simulink model "WPTwithMOTOR"  (R2021a)
settings: Solver=FixedStepDiscrete  StartTime=0.0  StopTime=Tfinal  FixedStep=SampleTime  RelTol=1e-3
InitFcn:
  | param
values from neighbouring files (symbols this model uses):
  Cp = 28.5e-9    (= 2.85e-08)    [param.m]
  Cs = 115e-9    (= 1.15e-07)    [param.m]
  ESRA = 1e-7    (= 1e-07)    [param.m]
  J = 0.001    [param.m]
  Lmotor = 1e-3    (= 0.001)    [param.m]
  Lp = 205e-6    (= 0.000205)    [param.m]
  Ls = 51e-6    (= 5.1e-05)    [param.m]
  M = 41e-6    (= 4.1e-05)    [param.m]
  RL = 40    [param.m]
  Rmotor = 2    [param.m]
  SampleTime = 1e-9    (= 1e-09)    [param.m]
  Tfinal = 0.1    [param.m]
  TL = 5    [param.m]
  VDC = 100    [param.m]
undefined symbols (not defined in the file or in its folder): ESLA
libraries: spsSeriesRLCBranchLib x13, spsVoltageMeasurementLib x10, spsCurrentMeasurementLib x10, spsMosfetLib x4, eeStairGenerator x3, spsFourierLib x2, spsDCVoltageSourceLib x1, spsDCMachineLib x1, spsTriangleGeneratorLib x1, spsVariableResistorLib x1, spspowerguiLib x1
settings Model: Creator=enes_  LastModifiedBy=enes_
settings SolverCC: AlgebraicLoopSolver=TrustRegion
settings DataIOCC: ReturnWorkspaceOutputs=off
settings DebuggingCC: SFMachineParentedDataDiag=warning  ArithmeticOperatorsInVariantConditions=warning
settings SFSimCC: SimUseLocalCustomCode=off  CustomCodeUndefinedFunction=UseInterfaceOnly
settings RTWCC: RTWUseLocalCustomCode=off

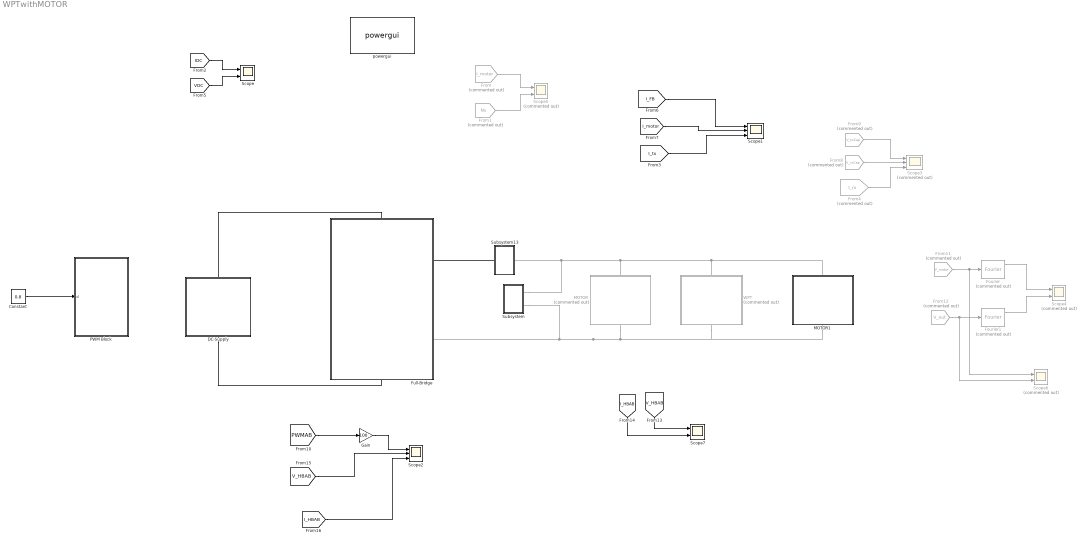
== system WPTwithMOTOR ==
  Constant : Constant  Value=0.8
  DC-Supply : Subsystem
  Fourier : spsFourierLib/Fourier  Commented=on  Freq=80e3  n=1  InInit=[0, 0]  Ts=SampleTime
      settings: SourceProductBaseCode=PS
  Fourier1 : spsFourierLib/Fourier  Commented=on  Freq=80e3  n=1  InInit=[0, 0]  Ts=SampleTime
      settings: SourceProductBaseCode=PS
  From : From  Commented=on  GotoTag=I_motor  TagVisibility=global
  From1 : From  Commented=on  GotoTag=Ns  TagVisibility=global
  From11 : From  Commented=on  GotoTag=V_motor  TagVisibility=global
  From12 : From  Commented=on  GotoTag=V_out  TagVisibility=global
  From4 : From  Commented=on  GotoTag=I_rx  TagVisibility=global
  From8 : From  Commented=on  GotoTag=V_rxCap  TagVisibility=global
  From9 : From  Commented=on  GotoTag=V_txCap  TagVisibility=global
  Full-Bridge : Subsystem
      settings: PortSchema="{\"entries\":[{\"content\":{\"sides\":[{\"content\":{\"connectorIds\":[]},\"type\":\"ConnectorPlacement.EquallySpacedRectSide\",\"uuid\":\"92c2640b-bb56-47f8-9c41-2323b38839f8\"},{\"content\":{\"connectorIds\":[\"RConn1\",\"RConn2\"],\"side\":\"RIGHT\"},\"type\":\"ConnectorPlacement.EquallySpacedRectSide\",\"uuid\":\"0b5c90a1-e2e1-4478-84c9-834496a6568e\"},{\"content\":{\"connectorIds\":[\"LConn1\"],\"side\":\"TOP\"},\"type\":\"ConnectorPlacement.EquallySpacedRectSide\",\"uuid\":\"1c803fb0-9096-4a7d-b495-aabd35d72306\"},{\"content\":{\"connectorIds\":[\"RConn3\"],\"side\":\"BOTTOM\"},\"type\":\"ConnectorPlacement.EquallySpacedRectSide\",\"uuid\":\"5a2d766c-8c3f-4943-ab0f-0e1988e2f8d8\"},{\"content\":{\"connectorIds\":[],\"side\":\"HIDDEN\"},\"type\":\"ConnectorPlacement.EquallySpacedRectSide\",\"uuid\":\"8868c32c-a67f-4887-a91d-dc24242eaee2\"}]},\"type\":\"ConnectorPlacement.EquallySpacedConnector\",\"uuid\":\"a3546067-6216-40b0-bae0-9d71271c5112\"}],\"packageUris\":[\"http://schema.mathworks.com/mf0/Connector/R2020b\"],\"version\":\"1.0\"}"
  Gain : Gain  Gain=100
  MOTOR : Subsystem  Commented=on
  MOTOR1 : Subsystem
  PWM Block : Subsystem
  Scope : Scope  NumInputPorts=2
  Scope1 : Scope  NumInputPorts=3
  Scope2 : Scope  NumInputPorts=3
  Scope3 : Scope  Commented=on  NumInputPorts=3
  Scope4 : Scope  Commented=on  NumInputPorts=2
  Scope5 : Scope  Commented=on  NumInputPorts=2
  Scope6 : Scope  Commented=on  NumInputPorts=2
  Scope7 : Scope  NumInputPorts=2
  Subsystem : Subsystem
  Subsystem13 : Subsystem
  WPT : Subsystem  Commented=on
  powergui : spspowerguiLib/powergui  Priority=1  SimulationMode=Discrete  SampleTime=SampleTime  frequency=60  Iterations=50  frequencyindice=0  Pbase=100e6  ErrMax=1e-4  UnitsV=kV  UnitsW=MW  buscounter=0  FunctionMessages=off  echomessages=off  EnableUseOfTLC=off  CurrentSourceSwitches=off  DisableSnubberDevices=off  DisableRonSwitches=off  DisableVfSwitches=off  DisplayEquations=off  AutomaticDiscreteSolvers=off  SolverType=Tustin/Backward Euler (TBE)  Interpol=off  ExternalGateDelay=off  methode=off  Ts=100  x0status=blocks  SPID=on  SwTol=0  HookPort=off  NonlinearTolerance=1e-4  nMaxIteration=100  ContinueOnMaxIteration=off  RestoreLinks=warning  ResistiveCurrentMeasurement=off  Frange=[1e3:1e3:240e3]  Ylog=off  Xlog=on  ShowGrid=off  save=off  variable=ZData  structure=inputVoltage  ZoomFFT=off  StartTime=0.0  cycles=100  DisplayStyle=1  fundamental=80000  FreqAxis=off  MaxFrequency=240e3  frequencyindicesteady=1  RmsSteady=1  display=off
  wires:
  [IDC] -> Scope/1
  [VDC] -> Scope/2
  From/1 -> Scope5/1
  From1/1 -> Scope5/2
  [I_FB] -> Scope1/1
  [I_motor] -> Scope1/2
  [I_tx] -> Scope1/3
  From9/1 -> Scope3/1
  From8/1 -> Scope3/2
  From4/1 -> Scope3/3
  From11/1 -> Scope6/1, Fourier/1
  From12/1 -> Scope6/2, Fourier1/1
  Fourier/1 -> Scope4/1
  Fourier1/1 -> Scope4/2
  Constant/1 -> PWM Block/1(d)
  [V_HBAB] -> Scope7/1
  [I_HBAB] -> Scope7/2
  [PWMAB] -> Gain/1
  [V_HBAB] -> Scope2/2
  Gain/1 -> Scope2/1
  [I_HBAB] -> Scope2/3
  connections:
  WPT/LConn1 -- Subsystem13/LConn1 -- Subsystem/LConn1 -- MOTOR/LConn1 -- MOTOR1/LConn1
  MOTOR/RConn1 -- Full-Bridge/RConn2 -- Subsystem/LConn2 -- WPT/RConn1 -- MOTOR1/RConn1
  Subsystem13/RConn1 -- Full-Bridge/RConn1
  DC-Supply/LConn1 -- Full-Bridge/LConn1
  DC-Supply/RConn1 -- Full-Bridge/RConn3

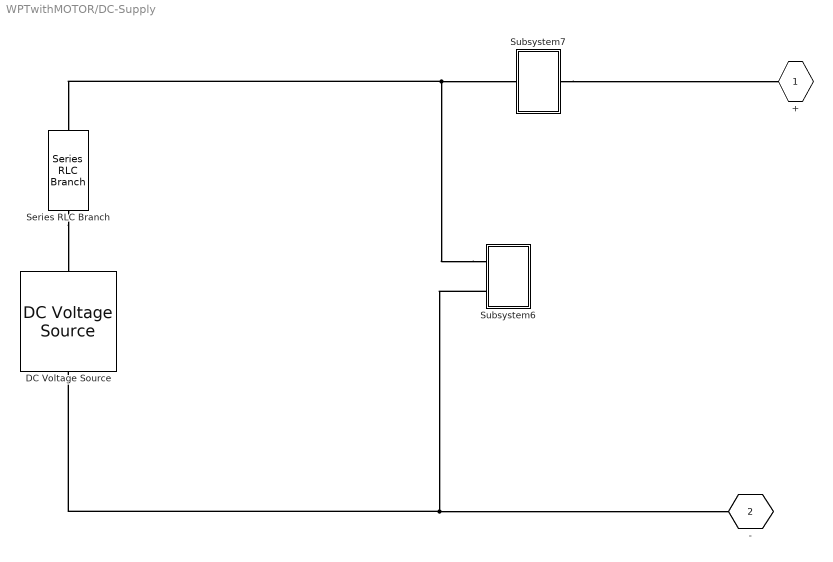
== system WPTwithMOTOR/DC-Supply ==
  DC Voltage Source : spsDCVoltageSourceLib/DC Voltage Source  Amplitude=VDC  Measurements=None
  Series RLC Branch : spsSeriesRLCBranchLib/Series RLC Branch  LConnTagsString=__new0  RConnTagsString=__new0  BranchType=RL  Resistance=1e-3  Inductance=1e-7  SetiL0=off  InitialCurrent=0  Capacitance=1e-6  Setx0=off  InitialVoltage=0  Measurements=None
  Subsystem6 : Subsystem
  Subsystem7 : Subsystem
  + : PMIOPort  Side=Left
  - : PMIOPort  Port=2  Side=Right
  connections:
  Subsystem6/LConn2 -- DC Voltage Source/LConn1 -- -/RConn1
  Subsystem6/LConn1 -- Series RLC Branch/LConn1 -- Subsystem7/RConn1
  Subsystem7/LConn1 -- +/RConn1
  Series RLC Branch/RConn1 -- DC Voltage Source/RConn1

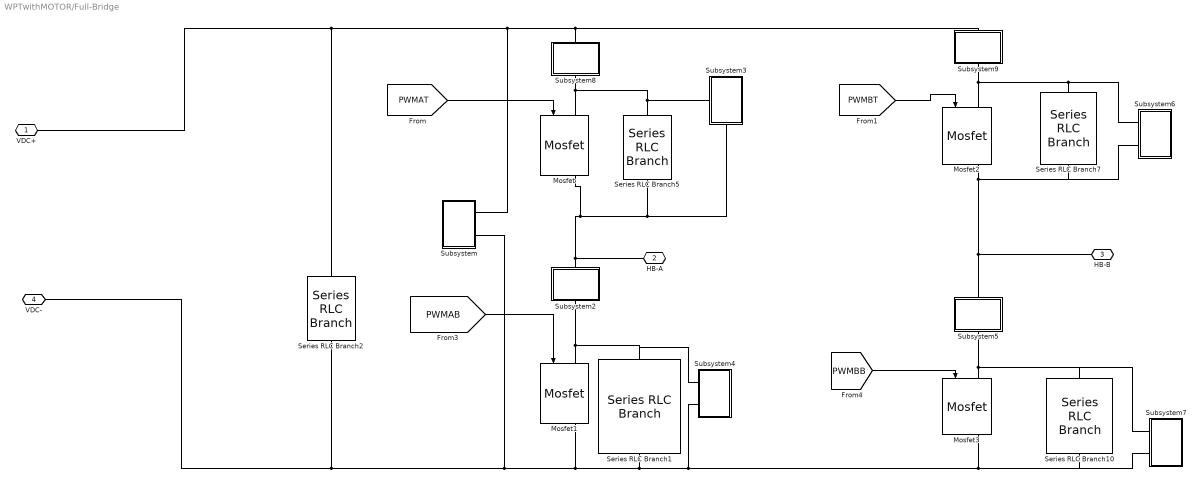
== system WPTwithMOTOR/Full-Bridge ==
  Mosfet{,1..3} (4 alike) : spsMosfetLib/Mosfet  Ron=0.1  Lon=0  Rd=0.01  Vfd=0  IC=0  Rs=1e5  Cs=inf  Measurements=on
  Series RLC Branch{1,5,7,10} (4 alike) : spsSeriesRLCBranchLib/Series RLC Branch  LConnTagsString=__new0  RConnTagsString=__new0  BranchType=C  Resistance=ESRA  Inductance=ESLA  SetiL0=off  InitialCurrent=0  Capacitance=10e-9  Setx0=off  InitialVoltage=0  Measurements=None
  Series RLC Branch2 : spsSeriesRLCBranchLib/Series RLC Branch  LConnTagsString=__new0  RConnTagsString=__new0  BranchType=C  Resistance=ESRA  Inductance=ESLA  SetiL0=off  InitialCurrent=0  Capacitance=100e-3  Setx0=off  InitialVoltage=0  Measurements=None
  Subsystem : Subsystem
  Subsystem2 : Subsystem
  Subsystem3 : Subsystem
      settings: PortSchema="{\"entries\":[{\"content\":{\"sides\":[{\"content\":{\"connectorIds\":[\"LConn1\"]},\"type\":\"ConnectorPlacement.EquallySpacedRectSide\",\"uuid\":\"5fd3471b-77c4-4add-974d-2088884e4e8f\"},{\"content\":{\"connectorIds\":[],\"side\":\"RIGHT\"},\"type\":\"ConnectorPlacement.EquallySpacedRectSide\",\"uuid\":\"3ed3d87c-239d-4488-bb47-dd20adb66433\"},{\"content\":{\"connectorIds\":[],\"side\":\"TOP\"},\"type\":\"ConnectorPlacement.EquallySpacedRectSide\",\"uuid\":\"7d1a83a5-f952-4011-a8a9-3e03fc6b2605\"},{\"content\":{\"connectorIds\":[\"RConn1\"],\"side\":\"BOTTOM\"},\"type\":\"ConnectorPlacement.EquallySpacedRectSide\",\"uuid\":\"37159049-9de9-498e-a62d-c9d42e905d7f\"}]},\"type\":\"ConnectorPlacement.EquallySpacedConnector\",\"uuid\":\"187da425-f362-4fb5-84e5-b88eb8acd0b2\"}],\"packageUris\":[\"http://schema.mathworks.com/mf0/Connector/R2020b\"],\"version\":\"1.0\"}"
  Subsystem4 : Subsystem
  Subsystem5 : Subsystem
  Subsystem6 : Subsystem
  Subsystem7 : Subsystem
  Subsystem8 : Subsystem
  Subsystem9 : Subsystem
  VDC+ : PMIOPort  Side=Left
  HB-A : PMIOPort  Port=2  Side=Right
  HB-B : PMIOPort  Port=3  Side=Right
  VDC- : PMIOPort  Port=4  Side=Right
  wires:
  [PWMAB] -> Mosfet1/1
  [PWMAT] -> Mosfet/1
  [PWMBB] -> Mosfet3/1
  [PWMBT] -> Mosfet2/1
  connections:
  Mosfet1/LConn1 -- Subsystem2/LConn1 -- Subsystem4/LConn1 -- Series RLC Branch1/LConn1
  Subsystem9/LConn1 -- Subsystem6/LConn1 -- Series RLC Branch7/LConn1 -- Mosfet2/LConn1
  VDC+/RConn1 -- Series RLC Branch2/LConn1 -- Subsystem/LConn1 -- Subsystem8/RConn1 -- Subsystem9/RConn1
  Series RLC Branch5/LConn1 -- Subsystem8/LConn1 -- Mosfet/LConn1 -- Subsystem3/LConn1
  VDC-/RConn1 -- Series RLC Branch2/RConn1 -- Subsystem/LConn2 -- Subsystem4/LConn2 -- Subsystem7/LConn2 -- Series RLC Branch10/RConn1 -- Mosfet3/RConn1 -- Series RLC Branch1/RConn1 -- Mosfet1/RConn1
  Subsystem6/LConn2 -- Series RLC Branch7/RConn1 -- HB-B/RConn1 -- Subsystem5/RConn1 -- Mosfet2/RConn1
  Subsystem3/RConn1 -- HB-A/RConn1 -- Subsystem2/RConn1 -- Mosfet/RConn1 -- Series RLC Branch5/RConn1
  Mosfet3/LConn1 -- Subsystem5/LConn1 -- Subsystem7/LConn1 -- Series RLC Branch10/LConn1

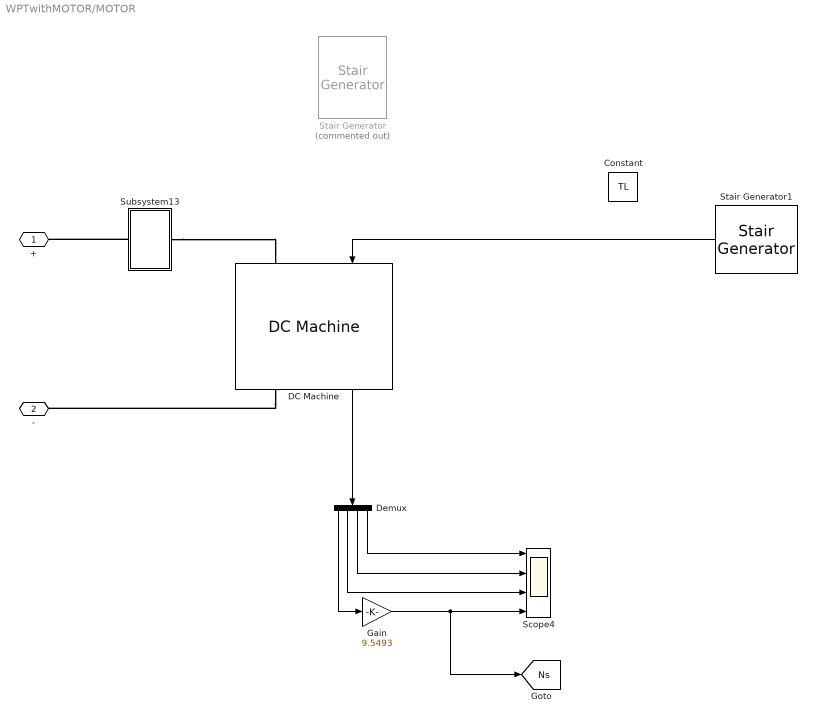
== system WPTwithMOTOR/MOTOR ==
  Constant : Constant  Value=TL
  DC Machine : spsDCMachineLib/DC Machine  PresetModel=No  MechanicalLoad=Torque TL  FieldType=Permanent magnet  ShowDetailedParameters=on  MeasurementBus=off  RLa="[ Rmotor  Lmotor]"  RLf="[ 240  120]"  Laf=1.8  MachineConstant=Back-emf constant (V/rpm)  Ke=Kf  Kt=1.8  J=J  Bm=Bm  Tf=Tf  w0=w0  Ifinit=1  TsPowergui=0  TsBlock=-1
  Demux : Demux
  Gain : Gain  Gain=9.5493
  Scope4 : Scope  NumInputPorts=4
  Stair Generator : eeStairGenerator/Stair Generator  Commented=on  LabelModeActiveChoice=Discrete  TimeInput=Tfinal*[0 1/3 2/3]  AmplitudeInput=TL*[0 1 1/2 ]  SampleTime=-1  RepeatPattern=off  OutDataTypeStr=double
      settings: SourceProductBaseCode=PS
  Stair Generator1 : eeStairGenerator/Stair Generator  LabelModeActiveChoice=Discrete  TimeInput=Tfinal*[0 1/4 2/4 3/4 ]  AmplitudeInput="TL*[1  0.5  1  0.6 ]"  SampleTime=SampleTime  RepeatPattern=off  OutDataTypeStr=double
      settings: SourceProductBaseCode=PS
  Subsystem13 : Subsystem
  + : PMIOPort  Side=Left
  - : PMIOPort  Port=2  Side=Right
  tag scope: Ns=global
  wires:
  Demux/2 -> Scope4/3
  Gain/1 -> [Ns], Scope4/4
  Demux/3 -> Scope4/2
  Demux/1 -> Gain/1
  Demux/4 -> Scope4/1
  DC Machine/1 -> Demux/1
  Stair Generator1/1 -> DC Machine/1
  connections:
  DC Machine/RConn1 -- -/RConn1
  Subsystem13/LConn1 -- DC Machine/LConn1
  Subsystem13/RConn1 -- +/RConn1

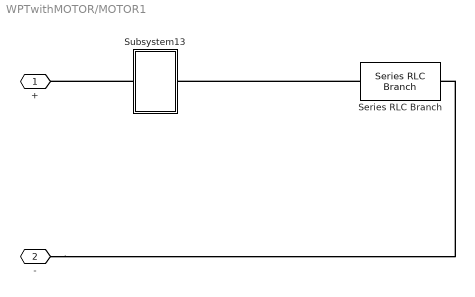
== system WPTwithMOTOR/MOTOR1 ==
  Series RLC Branch : spsSeriesRLCBranchLib/Series RLC Branch  LConnTagsString=__new0  RConnTagsString=__new0  BranchType=RL  Resistance=5  Inductance=7e-3  SetiL0=off  InitialCurrent=0  Capacitance=1e-6  Setx0=off  InitialVoltage=0  Measurements=None
  Subsystem13 : Subsystem
  + : PMIOPort  Side=Left
  - : PMIOPort  Port=2  Side=Right
  connections:
  Subsystem13/RConn1 -- +/RConn1
  Series RLC Branch/LConn1 -- Subsystem13/LConn1
  -/RConn1 -- Series RLC Branch/RConn1

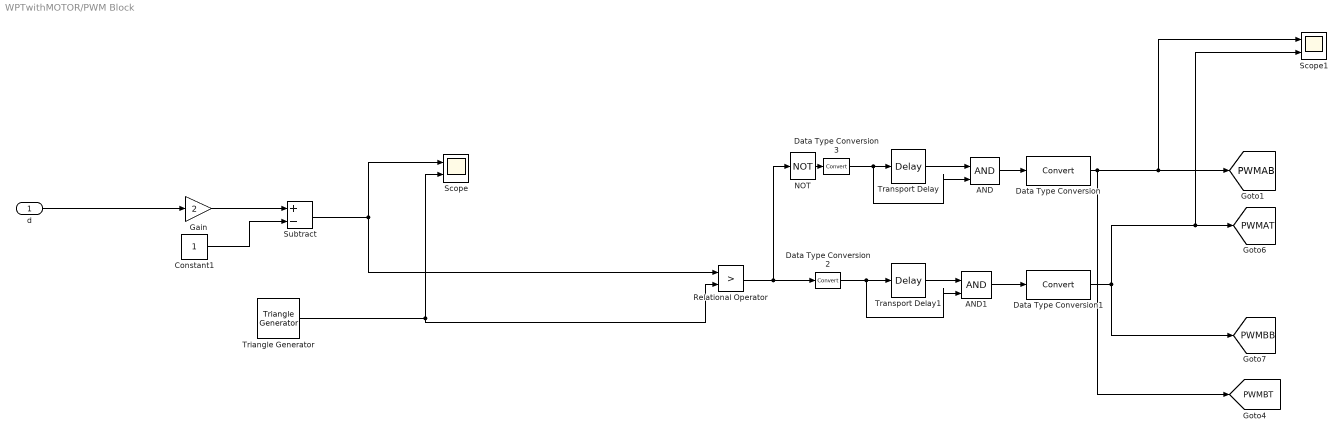
== system WPTwithMOTOR/PWM Block ==
  d : Inport
  AND : Logic  IconShape=distinctive  AllPortsSameDT=off  OutDataTypeStr=boolean
  AND1 : Logic  IconShape=distinctive  AllPortsSameDT=off  OutDataTypeStr=boolean
  Constant1 : Constant
  Data Type Conversion{,1..3} (4 alike) : DataTypeConversion
  Gain : Gain  Gain=2
  NOT : Logic  Operator=NOT  IconShape=distinctive  AllPortsSameDT=off  OutDataTypeStr=boolean
  Relational Operator : RelationalOperator  Operator=>  OutDataTypeStr=boolean  RndMeth=Simplest
  Scope : Scope  NumInputPorts=2
  Scope1 : Scope  NumInputPorts=2
  Subtract : Sum  Inputs=+-
  Transport Delay : TransportDelay  DelayTime=100e-9
  Transport Delay1 : TransportDelay  DelayTime=100e-9
  Triangle Generator : spsTriangleGeneratorLib/Triangle Generator  Freq=fsw  Phase=0  Ts=0
  tag scope: PWMAB=global, PWMAT=global, PWMBB=global, PWMBT=global
  wires:
  Triangle Generator/1 -> Relational Operator/2, Scope/2
  d/1 -> Gain/1
  Gain/1 -> Subtract/1
  Constant1/1 -> Subtract/2
  Subtract/1 -> Scope/1, Relational Operator/1
  Transport Delay/1 -> AND/1
  AND/1 -> Data Type Conversion/1
  Transport Delay1/1 -> AND1/1
  Relational Operator/1 -> Data Type Conversion2/1, NOT/1
  AND1/1 -> Data Type Conversion1/1
  Data Type Conversion/1 -> [PWMBT], Scope1/1, [PWMAB]
  Data Type Conversion1/1 -> [PWMBB], Scope1/2, [PWMAT]
  Data Type Conversion2/1 -> Transport Delay1/1, AND1/2
  NOT/1 -> Data Type Conversion3/1
  Data Type Conversion3/1 -> AND/2, Transport Delay/1

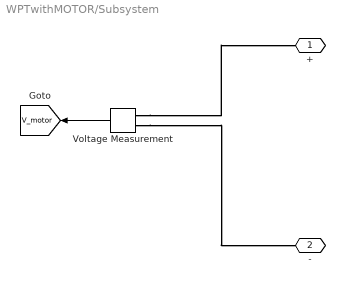
== system WPTwithMOTOR/Subsystem ==
  Voltage Measurement : spsVoltageMeasurementLib/Voltage Measurement  PhasorSimulation=off  OutputType=Complex  PSBequivalent=0
  + : PMIOPort  Side=Left
  - : PMIOPort  Port=2  Side=Left
  tag scope: V_motor=global
  wires:
  Voltage Measurement/1 -> [V_motor]
  connections:
  Voltage Measurement/LConn1 -- +/RConn1
  Voltage Measurement/LConn2 -- -/RConn1

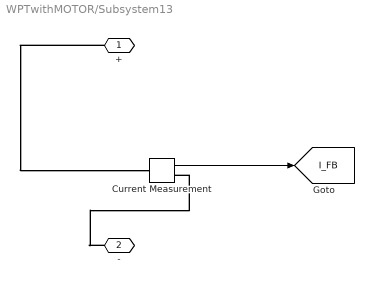
== system WPTwithMOTOR/Subsystem13 ==
  Current Measurement : spsCurrentMeasurementLib/Current Measurement  PhasorSimulation=off  OutputType=Complex  PSBequivalent=0
  + : PMIOPort  Side=Right
  - : PMIOPort  Port=2  Side=Left
  tag scope: I_FB=global
  wires:
  Current Measurement/1 -> [I_FB]
  connections:
  +/RConn1 -- Current Measurement/LConn1
  -/RConn1 -- Current Measurement/RConn1

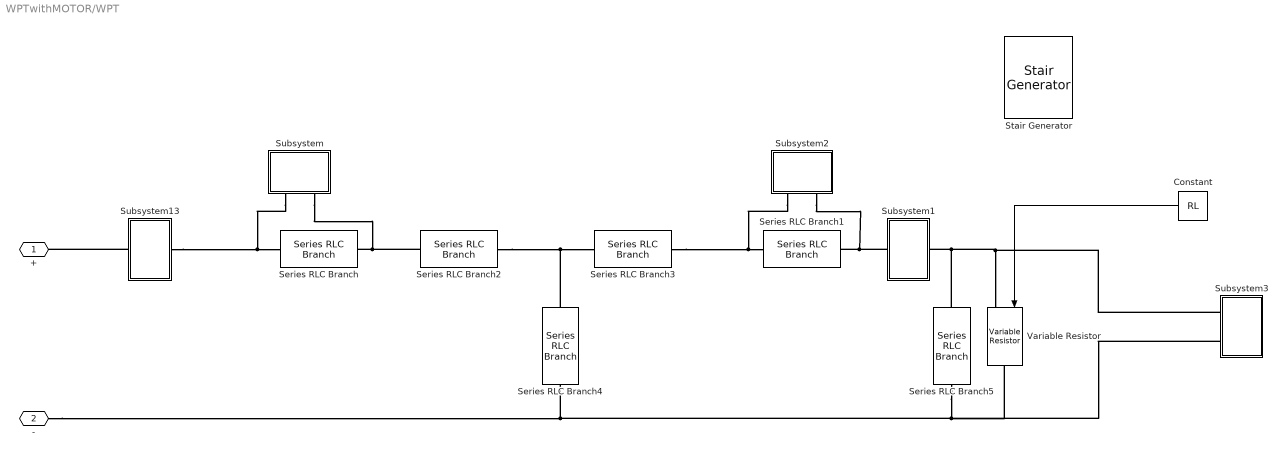
== system WPTwithMOTOR/WPT ==
  Constant : Constant  Value=RL
  Series RLC Branch : spsSeriesRLCBranchLib/Series RLC Branch  LConnTagsString=__new0  RConnTagsString=__new0  BranchType=C  Resistance=1  Inductance=1e-3  SetiL0=off  InitialCurrent=0  Capacitance=Cp  Setx0=off  InitialVoltage=0  Measurements=None
  Series RLC Branch1 : spsSeriesRLCBranchLib/Series RLC Branch  LConnTagsString=__new0  RConnTagsString=__new0  BranchType=C  Resistance=1  Inductance=1e-3  SetiL0=off  InitialCurrent=0  Capacitance=Cs  Setx0=off  InitialVoltage=0  Measurements=None
  Series RLC Branch2 : spsSeriesRLCBranchLib/Series RLC Branch  LConnTagsString=__new0  RConnTagsString=__new0  BranchType=L  Resistance=1  Inductance=Lp-M  SetiL0=off  InitialCurrent=0  Capacitance=Cp  Setx0=off  InitialVoltage=0  Measurements=None
  Series RLC Branch3 : spsSeriesRLCBranchLib/Series RLC Branch  LConnTagsString=__new0  RConnTagsString=__new0  BranchType=L  Resistance=1  Inductance=Ls-M  SetiL0=off  InitialCurrent=0  Capacitance=Cp  Setx0=off  InitialVoltage=0  Measurements=None
  Series RLC Branch4 : spsSeriesRLCBranchLib/Series RLC Branch  LConnTagsString=__new0  RConnTagsString=__new0  BranchType=L  Resistance=1  Inductance=Lp-M  SetiL0=off  InitialCurrent=0  Capacitance=Cp  Setx0=off  InitialVoltage=0  Measurements=None
  Series RLC Branch5 : spsSeriesRLCBranchLib/Series RLC Branch  LConnTagsString=__new0  RConnTagsString=__new0  BranchType=R  Resistance=1e6  Inductance=Ls-M  SetiL0=off  InitialCurrent=0  Capacitance=Cp  Setx0=off  InitialVoltage=0  Measurements=None
  Stair Generator : eeStairGenerator/Stair Generator  LabelModeActiveChoice=Discrete  TimeInput=Tfinal*[0 1/4 2/4 3/4 ]  AmplitudeInput=RL*[1 4 0 100 ]  SampleTime=-1  RepeatPattern=off  OutDataTypeStr=double
      settings: SourceProductBaseCode=PS
  Subsystem : Subsystem
  Subsystem1 : Subsystem
  Subsystem13 : Subsystem
  Subsystem2 : Subsystem
  Subsystem3 : Subsystem
  Variable Resistor : spsVariableResistorLib/Variable Resistor  Rabsmin=1e-3
      settings: SourceProductBaseCode=PS
  + : PMIOPort  Side=Left
  - : PMIOPort  Port=2  Side=Right
  wires:
  Constant/1 -> Variable Resistor/1
  connections:
  -/RConn1 -- Series RLC Branch5/RConn1 -- Subsystem3/LConn2 -- Variable Resistor/RConn1 -- Series RLC Branch4/RConn1
  Subsystem13/LConn1 -- Subsystem/LConn1 -- Series RLC Branch/LConn1
  Subsystem13/RConn1 -- +/RConn1
  Series RLC Branch2/LConn1 -- Subsystem/LConn2 -- Series RLC Branch/RConn1
  Series RLC Branch3/RConn1 -- Subsystem2/LConn1 -- Series RLC Branch1/RConn1
  Series RLC Branch4/LConn1 -- Series RLC Branch2/RConn1 -- Series RLC Branch3/LConn1
  Subsystem3/LConn1 -- Series RLC Branch5/LConn1 -- Subsystem1/LConn1 -- Variable Resistor/LConn1
  Subsystem1/RConn1 -- Subsystem2/LConn2 -- Series RLC Branch1/LConn1

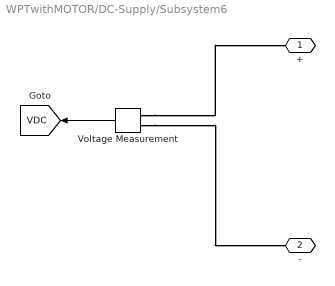
== system WPTwithMOTOR/DC-Supply/Subsystem6 ==
  Voltage Measurement : spsVoltageMeasurementLib/Voltage Measurement  PhasorSimulation=off  OutputType=Complex  PSBequivalent=0
  + : PMIOPort  Side=Left
  - : PMIOPort  Port=2  Side=Left
  tag scope: VDC=global
  wires:
  Voltage Measurement/1 -> [VDC]
  connections:
  Voltage Measurement/LConn1 -- +/RConn1
  Voltage Measurement/LConn2 -- -/RConn1

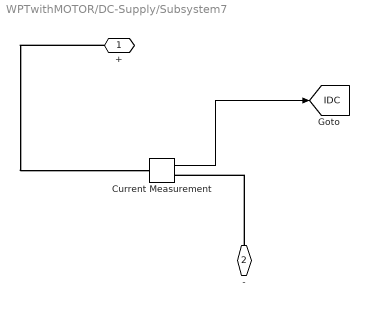
== system WPTwithMOTOR/DC-Supply/Subsystem7 ==
  Current Measurement : spsCurrentMeasurementLib/Current Measurement  PhasorSimulation=off  OutputType=Complex  PSBequivalent=0
  + : PMIOPort  Side=Right
  - : PMIOPort  Port=2  Side=Left
  tag scope: IDC=global
  wires:
  Current Measurement/1 -> [IDC]
  connections:
  +/RConn1 -- Current Measurement/LConn1
  -/RConn1 -- Current Measurement/RConn1

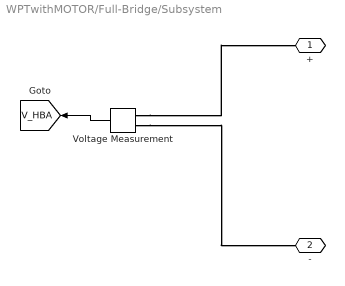
== system WPTwithMOTOR/Full-Bridge/Subsystem ==
  Voltage Measurement : spsVoltageMeasurementLib/Voltage Measurement  PhasorSimulation=off  OutputType=Complex  PSBequivalent=0
  + : PMIOPort  Side=Left
  - : PMIOPort  Port=2  Side=Left
  tag scope: V_HBA=global
  wires:
  Voltage Measurement/1 -> [V_HBA]
  connections:
  Voltage Measurement/LConn1 -- +/RConn1
  Voltage Measurement/LConn2 -- -/RConn1

== system WPTwithMOTOR/Full-Bridge/Subsystem2 ==
  Current Measurement : spsCurrentMeasurementLib/Current Measurement  PhasorSimulation=off  OutputType=Complex  PSBequivalent=0
  + : PMIOPort  Side=Right
  - : PMIOPort  Port=2  Side=Left
  tag scope: I_HBAB=global
  wires:
  Current Measurement/1 -> [I_HBAB]
  connections:
  +/RConn1 -- Current Measurement/LConn1
  -/RConn1 -- Current Measurement/RConn1

== system WPTwithMOTOR/Full-Bridge/Subsystem3 ==
  Voltage Measurement : spsVoltageMeasurementLib/Voltage Measurement  PhasorSimulation=off  OutputType=Complex  PSBequivalent=0
  + : PMIOPort  Side=Left
  - : PMIOPort  Port=2  Side=Right
  tag scope: V_HBAT=global
  wires:
  Voltage Measurement/1 -> [V_HBAT]
  connections:
  Voltage Measurement/LConn1 -- +/RConn1
  Voltage Measurement/LConn2 -- -/RConn1

== system WPTwithMOTOR/Full-Bridge/Subsystem4 ==
  Voltage Measurement : spsVoltageMeasurementLib/Voltage Measurement  PhasorSimulation=off  OutputType=Complex  PSBequivalent=0
  + : PMIOPort  Side=Left
  - : PMIOPort  Port=2  Side=Left
  tag scope: V_HBAB=global
  wires:
  Voltage Measurement/1 -> [V_HBAB]
  connections:
  Voltage Measurement/LConn1 -- +/RConn1
  Voltage Measurement/LConn2 -- -/RConn1

== system WPTwithMOTOR/Full-Bridge/Subsystem5 ==
  Current Measurement : spsCurrentMeasurementLib/Current Measurement  PhasorSimulation=off  OutputType=Complex  PSBequivalent=0
  + : PMIOPort  Side=Right
  - : PMIOPort  Port=2  Side=Left
  tag scope: I_HBBB=global
  wires:
  Current Measurement/1 -> [I_HBBB]
  connections:
  +/RConn1 -- Current Measurement/LConn1
  -/RConn1 -- Current Measurement/RConn1

== system WPTwithMOTOR/Full-Bridge/Subsystem6 ==
  Voltage Measurement : spsVoltageMeasurementLib/Voltage Measurement  PhasorSimulation=off  OutputType=Complex  PSBequivalent=0
  + : PMIOPort  Side=Left
  - : PMIOPort  Port=2  Side=Left
  tag scope: V_HBBT=global
  wires:
  Voltage Measurement/1 -> [V_HBBT]
  connections:
  Voltage Measurement/LConn1 -- +/RConn1
  Voltage Measurement/LConn2 -- -/RConn1

== system WPTwithMOTOR/Full-Bridge/Subsystem7 ==
  Voltage Measurement : spsVoltageMeasurementLib/Voltage Measurement  PhasorSimulation=off  OutputType=Complex  PSBequivalent=0
  + : PMIOPort  Side=Left
  - : PMIOPort  Port=2  Side=Left
  tag scope: V_HBBB=global
  wires:
  Voltage Measurement/1 -> [V_HBBB]
  connections:
  Voltage Measurement/LConn1 -- +/RConn1
  Voltage Measurement/LConn2 -- -/RConn1

== system WPTwithMOTOR/Full-Bridge/Subsystem8 ==
  Current Measurement : spsCurrentMeasurementLib/Current Measurement  PhasorSimulation=off  OutputType=Complex  PSBequivalent=0
  + : PMIOPort  Side=Right
  - : PMIOPort  Port=2  Side=Left
  tag scope: I_HBA=global
  wires:
  Current Measurement/1 -> [I_HBA]
  connections:
  +/RConn1 -- Current Measurement/LConn1
  -/RConn1 -- Current Measurement/RConn1

== system WPTwithMOTOR/Full-Bridge/Subsystem9 ==
  Current Measurement : spsCurrentMeasurementLib/Current Measurement  PhasorSimulation=off  OutputType=Complex  PSBequivalent=0
  + : PMIOPort  Side=Right
  - : PMIOPort  Port=2  Side=Left
  tag scope: I_HBB=global
  wires:
  Current Measurement/1 -> [I_HBB]
  connections:
  +/RConn1 -- Current Measurement/LConn1
  -/RConn1 -- Current Measurement/RConn1

== system WPTwithMOTOR/MOTOR/Subsystem13 ==
  Current Measurement : spsCurrentMeasurementLib/Current Measurement  PhasorSimulation=off  OutputType=Complex  PSBequivalent=0
  + : PMIOPort  Side=Right
  - : PMIOPort  Port=2  Side=Left
  tag scope: I_motor=global
  wires:
  Current Measurement/1 -> [I_motor]
  connections:
  +/RConn1 -- Current Measurement/LConn1
  -/RConn1 -- Current Measurement/RConn1

== system WPTwithMOTOR/MOTOR1/Subsystem13 ==
  Current Measurement : spsCurrentMeasurementLib/Current Measurement  PhasorSimulation=off  OutputType=Complex  PSBequivalent=0
  + : PMIOPort  Side=Right
  - : PMIOPort  Port=2  Side=Left
  tag scope: I_motor=global
  wires:
  Current Measurement/1 -> [I_motor]
  connections:
  +/RConn1 -- Current Measurement/LConn1
  -/RConn1 -- Current Measurement/RConn1

== system WPTwithMOTOR/WPT/Subsystem ==
  Voltage Measurement : spsVoltageMeasurementLib/Voltage Measurement  PhasorSimulation=off  OutputType=Complex  PSBequivalent=0
  + : PMIOPort  Side=Left
  - : PMIOPort  Port=2  Side=Left
  tag scope: V_txCap=global
  wires:
  Voltage Measurement/1 -> [V_txCap]
  connections:
  Voltage Measurement/LConn1 -- +/RConn1
  Voltage Measurement/LConn2 -- -/RConn1

== system WPTwithMOTOR/WPT/Subsystem1 ==
  Current Measurement : spsCurrentMeasurementLib/Current Measurement  PhasorSimulation=off  OutputType=Complex  PSBequivalent=0
  + : PMIOPort  Side=Right
  - : PMIOPort  Port=2  Side=Left
  tag scope: I_rx=global
  wires:
  Current Measurement/1 -> [I_rx]
  connections:
  +/RConn1 -- Current Measurement/LConn1
  -/RConn1 -- Current Measurement/RConn1

== system WPTwithMOTOR/WPT/Subsystem13 ==
  Current Measurement : spsCurrentMeasurementLib/Current Measurement  PhasorSimulation=off  OutputType=Complex  PSBequivalent=0
  + : PMIOPort  Side=Right
  - : PMIOPort  Port=2  Side=Left
  tag scope: I_tx=global
  wires:
  Current Measurement/1 -> [I_tx]
  connections:
  +/RConn1 -- Current Measurement/LConn1
  -/RConn1 -- Current Measurement/RConn1

== system WPTwithMOTOR/WPT/Subsystem2 ==
  Voltage Measurement : spsVoltageMeasurementLib/Voltage Measurement  PhasorSimulation=off  OutputType=Complex  PSBequivalent=0
  + : PMIOPort  Side=Left
  - : PMIOPort  Port=2  Side=Left
  tag scope: V_rxCap=global
  wires:
  Voltage Measurement/1 -> [V_rxCap]
  connections:
  Voltage Measurement/LConn1 -- +/RConn1
  Voltage Measurement/LConn2 -- -/RConn1

== system WPTwithMOTOR/WPT/Subsystem3 ==
  Voltage Measurement : spsVoltageMeasurementLib/Voltage Measurement  PhasorSimulation=off  OutputType=Complex  PSBequivalent=0
  + : PMIOPort  Side=Left
  - : PMIOPort  Port=2  Side=Left
  tag scope: V_out=global
  wires:
  Voltage Measurement/1 -> [V_out]
  connections:
  Voltage Measurement/LConn1 -- +/RConn1
  Voltage Measurement/LConn2 -- -/RConn1
